simulink model "EL_Model_Simulink"  (R2022a)
settings: Solver=ode5  StartTime=0.0  StopTime=1  FixedStep=0.001  RelTol=1e-3
values from neighbouring files (symbols this model uses):
  a_joint = 160/180*pi    (= 2.79252680319)    [EL_Model_Activation.m]    (also in Form_Finding_Activation.m)
  C_damping = 150    [EL_Model_Activation.m]
  Gt = g'*G    [EL_Model_Activation.m]
  k_cable = 1200    [EL_Model_Activation.m]    (also in Form_Finding_Activation.m)
  k_joint = 35    [EL_Model_Activation.m]    (also in Form_Finding_Activation.m)
  l_cable = sqrt(6)/4*l_leg*sin(a_joint/2)*(1 - delta)    [EL_Model_Activation.m]    (also in Form_Finding_Activation.m = sqrt(6)/4*l_bar*sin(a_joint/2)*(1 - delta))
  l_leg = 0.30    (= 0.3)    [EL_Model_Activation.m]
  m_leg = density*(l_leg*pi*radius^2)+ m_motor + m_battery    (= 0.662767695314)    [EL_Model_Activation.m]
  mu_k = 0.4    [EL_Model_Activation.m]
  mu_s = 0.45    [EL_Model_Activation.m]
  nu_s = 0.25    [EL_Model_Activation.m]
  radius = 0.005    [EL_Model_Activation.m]
  T_damping = 10    [EL_Model_Activation.m]
  X = zeros(36,36,6)    [EL_Model_Activation.m]
  Xbark = zeros(3,36,6)    [EL_Model_Activation.m]
  Xk = zeros(3,36,6)    [EL_Model_Activation.m]
  Y = zeros(36,36,24)    [EL_Model_Activation.m]
  Yk = zeros(3,36,24)    [EL_Model_Activation.m]
settings Model: Creator=LZY-ALIENWARE15  LastModifiedBy=S2974177
settings SolverCC: ExtrapolationOrder=3  AlgebraicLoopSolver=TrustRegion
settings DebuggingCC: UnconnectedInputMsg=warning  UnconnectedOutputMsg=warning  UnconnectedLineMsg=warning  SFMachineParentedDataDiag=warning  UnderSpecifiedDimensionMsg=warning
settings RTWCC: DLArmComputeVersion=19.05

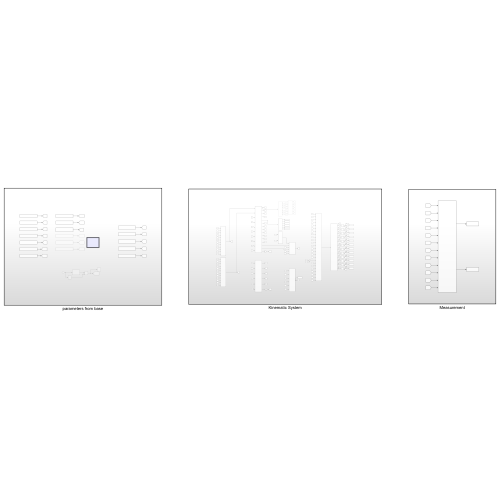
[thumbnail: Simulink's stored preview of the top-level diagram]
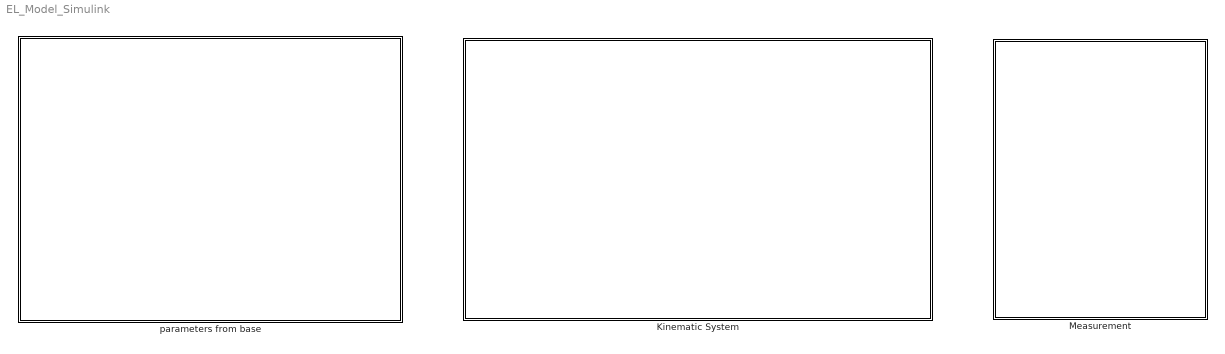
== system EL_Model_Simulink ==
  Kinematic System : Subsystem
  Measurement : Subsystem
  parameters from base : Subsystem

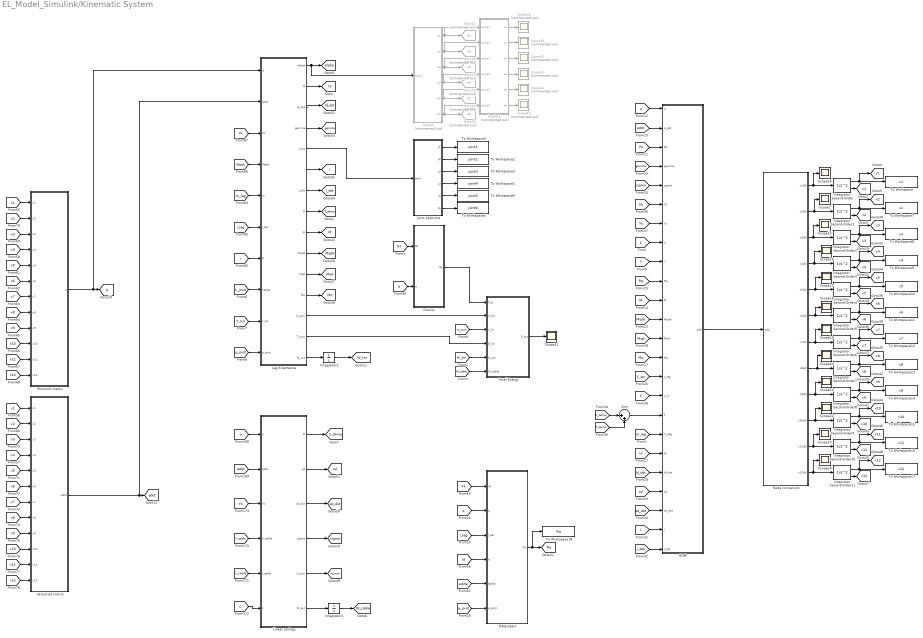
== system EL_Model_Simulink/Kinematic System ==
  Angles : MATLAB Function  Commented=on  TreatAsAtomicUnit=on
  Angles1 : MATLAB Function  Commented=on  TreatAsAtomicUnit=on
  D'Alembert : MATLAB Function  TreatAsAtomicUnit=on
  EOM : MATLAB Function  TreatAsAtomicUnit=on
  Goto13 : Goto  Commented=on  GotoTag=a1  TagVisibility=global
  Goto14 : Goto  Commented=on  GotoTag=a2  TagVisibility=global
  Goto15 : Goto  Commented=on  GotoTag=a3  TagVisibility=global
  Goto16 : Goto  Commented=on  GotoTag=a4  TagVisibility=global
  Goto17 : Goto  Commented=on  GotoTag=a5  TagVisibility=global
  Goto18 : Goto  Commented=on  GotoTag=a6  TagVisibility=global
  Gravity : MATLAB Function  TreatAsAtomicUnit=on
  "Integrator, Second-Order" : SecondOrderIntegrator  ICX=x1_ini  ICDXDT=v1_ini
  "Integrator, Second-Order1" : SecondOrderIntegrator  ICX=x2_ini  ICDXDT=v2_ini
  "Integrator, Second-Order10" : SecondOrderIntegrator  ICX=x11_ini  ICDXDT=v11_ini
  "Integrator, Second-Order11" : SecondOrderIntegrator  ICX=x12_ini  ICDXDT=v12_ini
  "Integrator, Second-Order2" : SecondOrderIntegrator  ICX=x3_ini  ICDXDT=v3_ini
  "Integrator, Second-Order3" : SecondOrderIntegrator  ICX=x4_ini  ICDXDT=v4_ini
  "Integrator, Second-Order4" : SecondOrderIntegrator  ICX=x5_ini  ICDXDT=v5_ini
  "Integrator, Second-Order5" : SecondOrderIntegrator  ICX=x6_ini  ICDXDT=v6_ini
  "Integrator, Second-Order6" : SecondOrderIntegrator  ICX=x7_ini  ICDXDT=v7_ini
  "Integrator, Second-Order7" : SecondOrderIntegrator  ICX=x8_ini  ICDXDT=v8_ini
  "Integrator, Second-Order8" : SecondOrderIntegrator  ICX=x9_ini  ICDXDT=v9_ini
  "Integrator, Second-Order9" : SecondOrderIntegrator  ICX=x10_ini  ICDXDT=v10_ini
  Integrator1 : Integrator
  Integrator2 : Integrator
  Joint positions : MATLAB Function  TreatAsAtomicUnit=on
  Leg Kinematics : MATLAB Function  TreatAsAtomicUnit=on
  Linear springs : MATLAB Function  TreatAsAtomicUnit=on
  Node conversion : MATLAB Function  TreatAsAtomicUnit=on
  Positions matrix : MATLAB Function  TreatAsAtomicUnit=on
  Scope{2,11,14..24} (13 alike) : Scope
  Scope{38..43} (6 alike) : Scope  Commented=on
  Sum : Sum  Inputs=|++
  To Workspace : ToWorkspace  VariableName=x1  SaveFormat=Timeseries  SampleTime=-1
  To Workspace1 : ToWorkspace  VariableName=joint4  SaveFormat=Timeseries  SampleTime=-1
  To Workspace10 : ToWorkspace  VariableName=x5  SaveFormat=Timeseries  SampleTime=-1
  To Workspace11 : ToWorkspace  VariableName=x6  SaveFormat=Timeseries  SampleTime=-1
  To Workspace12 : ToWorkspace  VariableName=x7  SaveFormat=Timeseries  SampleTime=-1
  To Workspace13 : ToWorkspace  VariableName=x8  SaveFormat=Timeseries  SampleTime=-1
  To Workspace14 : ToWorkspace  VariableName=x9  SaveFormat=Timeseries  SampleTime=-1
  To Workspace15 : ToWorkspace  VariableName=x10  SaveFormat=Timeseries  SampleTime=-1
  To Workspace16 : ToWorkspace  VariableName=x11  SaveFormat=Timeseries  SampleTime=-1
  To Workspace17 : ToWorkspace  VariableName=x12  SaveFormat=Timeseries  SampleTime=-1
  To Workspace18 : ToWorkspace  VariableName=Rq  SaveFormat=Timeseries  SampleTime=-1
  To Workspace2 : ToWorkspace  VariableName=joint2  SaveFormat=Timeseries  SampleTime=-1
  To Workspace3 : ToWorkspace  VariableName=joint3  SaveFormat=Timeseries  SampleTime=-1
  To Workspace4 : ToWorkspace  VariableName=joint1  SaveFormat=Timeseries  SampleTime=-1
  To Workspace5 : ToWorkspace  VariableName=joint6  SaveFormat=Timeseries  SampleTime=-1
  To Workspace6 : ToWorkspace  VariableName=joint5  SaveFormat=Timeseries  SampleTime=-1
  To Workspace7 : ToWorkspace  VariableName=x2  SaveFormat=Timeseries  SampleTime=-1
  To Workspace8 : ToWorkspace  VariableName=x3  SaveFormat=Timeseries  SampleTime=-1
  To Workspace9 : ToWorkspace  VariableName=x4  SaveFormat=Timeseries  SampleTime=-1
  Total Energy : MATLAB Function  TreatAsAtomicUnit=on
  Velocities matrix : MATLAB Function  TreatAsAtomicUnit=on
  tag scope: C_damp=global, I=global, I_dot=global, M=global, Mq=global, Mqd=global, Mqdd=global, Rq=global, T_damp=global, Vc_sum=global, W_cable=global, W_tor=global, alpha=global, gamma=global, ld=global, ld_dot=global, q=global, qdot=global, sd=global, sd_dot=global, sigma=global, v10=global, v11=global, v12=global, v1=global, v2=global, v3=global, v4=global, v5=global, v6=global, v7=global, v8=global, v9=global, x10=global, x11=global, x12=global, x1=global, x2=global, x3=global, x4=global, x5=global, x6=global, x7=global, x8=global, x9=global
  wires:
  [qdot] -> Linear springs/2(qdot)
  [Yk] -> Linear springs/3(Yk)
  [v7] -> Velocities matrix/7(v7)
  [x3] -> Positions matrix/3(x3)
  Joint positions/6(j6) -> To Workspace5/1
  [q] -> Linear springs/1(q)
  Angles/2(a2) -> Angles1/2(alpha2), Goto14/1
  [v10] -> Velocities matrix/10(v10)
  [C] -> Linear springs/6(c)
  Angles/6(a6) -> Angles1/6(alpha6), Goto18/1
  Joint positions/1(j1) -> To Workspace4/1
  Gravity/1(Vg) -> Total Energy/1(V_g)
  Angles/5(a5) -> Angles1/5(alpha5), Goto17/1
  Joint positions/2(j2) -> To Workspace2/1
  [x12] -> Positions matrix/12(x12)
  [m_leg] -> Leg Kinematics/5(m)
  [v6] -> Velocities matrix/6(v6)
  [v4] -> Velocities matrix/4(v4)
  [r] -> Leg Kinematics/7(R)
  [l_leg] -> Leg Kinematics/6(l_bar)
  [q] -> Gravity/2(q)
  Linear springs/5(V_sum) -> [Vc_sum]
  [x2] -> Positions matrix/2(x2)
  [v3] -> Velocities matrix/3(v3)
  Angles/4(a4) -> Angles1/4(alpha4), Goto16/1
  Angles/3(a3) -> Angles1/3(alpha3), Goto15/1
  Leg Kinematics/1(alpha) -> [alpha], Angles/1(alpha)
  [Xk] -> Leg Kinematics/3(Xk)
  Angles/1(a1) -> Goto13/1, Angles1/1(alpha1)
  [x5] -> Positions matrix/5(x5)
  Joint positions/3(j3) -> To Workspace3/1
  [Xbark] -> Leg Kinematics/4(Xbark)
  Leg Kinematics/5(joint) -> Joint positions/1(joint)
  Velocities matrix/1(qdot) -> Leg Kinematics/2(qdot), [qdot]
  [v11] -> Velocities matrix/11(v11)
  Positions matrix/1(q) -> Leg Kinematics/1(q), [q]
  [v9] -> Velocities matrix/9(v9)
  [l_cable] -> Linear springs/5(l_cable)
  [v8] -> Velocities matrix/8(v8)
  [v1] -> Velocities matrix/1(v1)
  [x6] -> Positions matrix/6(x6)
  [x1] -> Positions matrix/1(x1)
  [x7] -> Positions matrix/7(x7)
  [v5] -> Velocities matrix/5(v5)
  [x8] -> Positions matrix/8(x8)
  [k_cable] -> Linear springs/4(k_cable)
  [x11] -> Positions matrix/11(x11)
  [v2] -> Velocities matrix/2(v2)
  [v12] -> Velocities matrix/12(v12)
  Joint positions/5(j5) -> To Workspace6/1
  [x4] -> Positions matrix/4(x4)
  [x10] -> Positions matrix/10(x10)
  [x9] -> Positions matrix/9(x9)
  Joint positions/4(j4) -> To Workspace1/1
  Linear springs/1(D) -> [C_damp]
  Leg Kinematics/13(U_sum) -> Total Energy/2(V_tor)
  [C_tor] -> Leg Kinematics/9(c_tor)
  [k_joint] -> Leg Kinematics/8(kappa)
  [a_joint] -> Leg Kinematics/10(a_joint)
  [Vc_sum] -> Total Energy/3(V_lin)
  Total Energy/1(E_tot) -> Scope11/1
  Leg Kinematics/15(W_out) -> Integrator2/1
  Integrator1/1 -> [W_cable]
  Integrator2/1 -> [W_tor]
  Leg Kinematics/9(M) -> [M]
  [W_tor] -> Total Energy/5(W_tor)
  [W_cable] -> Total Energy/6(W_cable)
  Leg Kinematics/14(T_sum) -> Total Energy/4(E_kin)
  [Gt] -> Gravity/1(Gt)
  [X] -> EOM/8(X)
  [Y] -> EOM/9(Y)
  [sigma] -> EOM/5(sigma)
  Linear springs/4(sigma) -> [sigma]
  [Gt] -> EOM/3(Gt)
  [q] -> EOM/1(q)
  [qdot] -> EOM/2(q_dot)
  [M] -> EOM/11(M)
  Leg Kinematics/10(Mqdd) -> [Mqdd]
  Leg Kinematics/11(Mqd) -> [Mqd]
  Leg Kinematics/12(Mq) -> [Mq]
  [Mq] -> EOM/14(Mq)
  [Mqd] -> EOM/13(Mqd)
  [Mqdd] -> EOM/12(Mqdd)
  [Rq] -> EOM/10(Rq)
  Leg Kinematics/2(ld) -> [ld]
  Leg Kinematics/8(D) -> [T_damp]
  Linear springs/3(sd_dot) -> [sd_dot]
  Linear springs/2(sd) -> [sd]
  Leg Kinematics/3(ld_dot) -> [ld_dot]
  Leg Kinematics/4(gamma) -> [gamma]
  Leg Kinematics/7(I_dot) -> [I_dot]
  Leg Kinematics/6(I) -> [I]
  [m_leg] -> EOM/18(m_leg)
  [I_dot] -> EOM/24(I_dot)
  [I] -> EOM/23(I)
  [sd_dot] -> EOM/22(sd_dot)
  [sd] -> EOM/21(sd)
  [ld_dot] -> EOM/20(ld_dot)
  [ld] -> EOM/19(ld)
  [gamma] -> EOM/4(gamma)
  [C] -> EOM/16(c_lin)
  [C_tor] -> EOM/15(c_leg)
  [C_damp] -> Sum/1
  [T_damp] -> Sum/2
  Sum/1 -> EOM/17(f)
  [Xk] -> EOM/6(Xk)
  [Yk] -> EOM/7(Yk)
  Angles1/1(a1) -> Scope38/1
  Angles1/2(a2) -> Scope39/1
  Angles1/3(a3) -> Scope40/1
  Angles1/4(a4) -> Scope41/1
  Angles1/5(a5) -> Scope42/1
  Angles1/6(a6) -> Scope43/1
  Linear springs/6(W_out) -> Integrator1/1
  "Integrator, Second-Order10"/2 -> [v11]
  "Integrator, Second-Order9"/1 -> [x10], To Workspace15/1
  "Integrator, Second-Order5"/1 -> [x6], To Workspace11/1
  "Integrator, Second-Order5"/2 -> [v6]
  "Integrator, Second-Order10"/1 -> [x11], To Workspace16/1
  "Integrator, Second-Order8"/1 -> [x9], To Workspace14/1
  "Integrator, Second-Order4"/2 -> [v5]
  "Integrator, Second-Order7"/1 -> [x8], To Workspace13/1
  "Integrator, Second-Order2"/1 -> [x3], To Workspace8/1
  "Integrator, Second-Order1"/1 -> [x2], To Workspace7/1
  "Integrator, Second-Order3"/2 -> [v4]
  Node conversion/2(x2dd) -> "Integrator, Second-Order1"/1, Scope2/1
  "Integrator, Second-Order"/2 -> [v1]
  "Integrator, Second-Order1"/2 -> [v2]
  Node conversion/9(x9dd) -> Scope21/1, "Integrator, Second-Order8"/1
  Node conversion/10(x10dd) -> Scope22/1, "Integrator, Second-Order9"/1
  "Integrator, Second-Order"/1 -> [x1], To Workspace/1
  Node conversion/8(x8dd) -> Scope20/1, "Integrator, Second-Order7"/1
  Node conversion/3(x3dd) -> Scope15/1, "Integrator, Second-Order2"/1
  "Integrator, Second-Order3"/1 -> [x4], To Workspace9/1
  Node conversion/4(x4dd) -> Scope16/1, "Integrator, Second-Order3"/1
  "Integrator, Second-Order7"/2 -> [v8]
  "Integrator, Second-Order9"/2 -> [v10]
  Node conversion/7(x7dd) -> Scope19/1, "Integrator, Second-Order6"/1
  "Integrator, Second-Order8"/2 -> [v9]
  Node conversion/5(x5dd) -> Scope17/1, "Integrator, Second-Order4"/1
  "Integrator, Second-Order4"/1 -> [x5], To Workspace10/1
  "Integrator, Second-Order2"/2 -> [v3]
  "Integrator, Second-Order11"/1 -> [x12], To Workspace17/1
  Node conversion/1(x1dd) -> Scope14/1, "Integrator, Second-Order"/1
  "Integrator, Second-Order6"/2 -> [v7]
  Node conversion/12(x12dd) -> "Integrator, Second-Order11"/1, Scope24/1
  "Integrator, Second-Order11"/2 -> [v12]
  Node conversion/11(x11dd) -> Scope23/1, "Integrator, Second-Order10"/1
  Node conversion/6(x6dd) -> Scope18/1, "Integrator, Second-Order5"/1
  "Integrator, Second-Order6"/1 -> [x7], To Workspace12/1
  EOM/1(qdd) -> Node conversion/1(qdd)
  [q] -> D'Alembert/2(q)
  [a_joint] -> D'Alembert/6(a_joint)
  [alpha] -> D'Alembert/5(alpha)
  [l_leg] -> D'Alembert/3(l_bar)
  [ld] -> D'Alembert/4(d)
  D'Alembert/1(Rq) -> To Workspace18/1, [Rq]
  [Xk] -> D'Alembert/1(Xk)

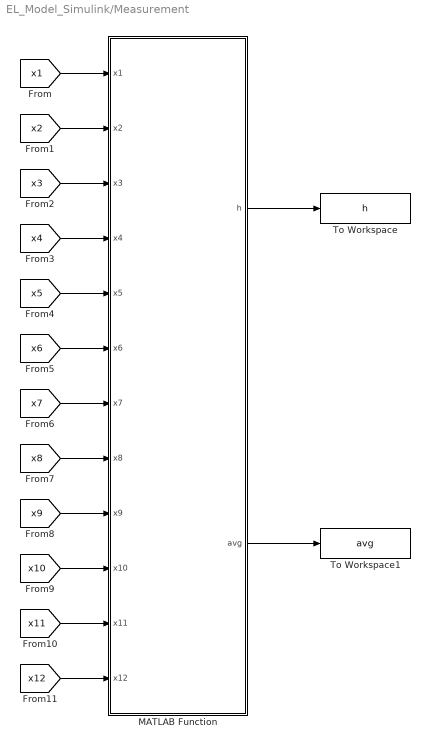
== system EL_Model_Simulink/Measurement ==
  MATLAB Function : MATLAB Function  TreatAsAtomicUnit=on
  To Workspace : ToWorkspace  VariableName=h  SaveFormat=Timeseries  SampleTime=-1
  To Workspace1 : ToWorkspace  VariableName=avg  SaveFormat=Timeseries  SampleTime=-1
  wires:
  [x1] -> MATLAB Function/1(x1)
  [x2] -> MATLAB Function/2(x2)
  [x3] -> MATLAB Function/3(x3)
  [x4] -> MATLAB Function/4(x4)
  [x5] -> MATLAB Function/5(x5)
  [x6] -> MATLAB Function/6(x6)
  [x8] -> MATLAB Function/8(x8)
  [x9] -> MATLAB Function/9(x9)
  [x10] -> MATLAB Function/10(x10)
  [x11] -> MATLAB Function/11(x11)
  [x12] -> MATLAB Function/12(x12)
  [x7] -> MATLAB Function/7(x7)
  MATLAB Function/1(h) -> To Workspace/1
  MATLAB Function/2(avg) -> To Workspace1/1

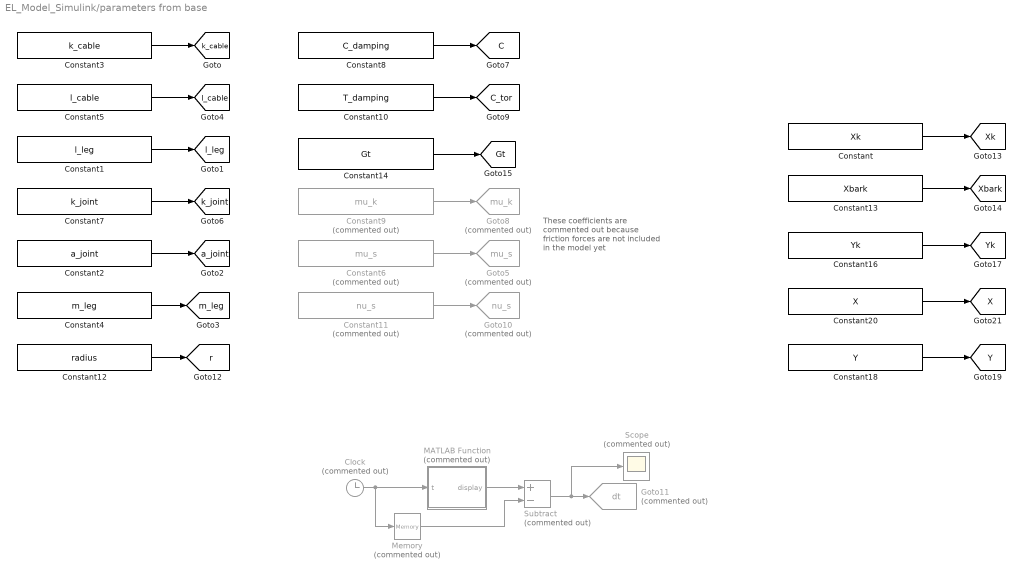
== system EL_Model_Simulink/parameters from base ==
  note: These coefficients
      | are commented
      | out because friction
      | forces are not
      | included in the
      | model yet
  Clock : Clock  Commented=on
  Constant : Constant  Value=Xk  VectorParams1D=off
  Constant1 : Constant  Value=l_leg
  Constant10 : Constant  Value=T_damping
  Constant11 : Constant  Commented=on  Value=nu_s
  Constant12 : Constant  Value=radius
  Constant13 : Constant  Value=Xbark  VectorParams1D=off
  Constant14 : Constant  Value=Gt
  Constant16 : Constant  Value=Yk  VectorParams1D=off
  Constant18 : Constant  Value=Y  VectorParams1D=off
  Constant2 : Constant  Value=a_joint
  Constant20 : Constant  Value=X  VectorParams1D=off
  Constant3 : Constant  Value=k_cable
  Constant4 : Constant  Value=m_leg
  Constant5 : Constant  Value=l_cable
  Constant6 : Constant  Commented=on  Value=mu_s
  Constant7 : Constant  Value=k_joint
  Constant8 : Constant  Value=C_damping
  Constant9 : Constant  Commented=on  Value=mu_k
  Goto10 : Goto  Commented=on  GotoTag=nu_s  TagVisibility=global
  Goto11 : Goto  Commented=on  GotoTag=dt  TagVisibility=global
  Goto5 : Goto  Commented=on  GotoTag=mu_s  TagVisibility=global
  Goto8 : Goto  Commented=on  GotoTag=mu_k  TagVisibility=global
  MATLAB Function : MATLAB Function  Commented=on  TreatAsAtomicUnit=on
  Memory : Memory  Commented=on
  Scope : Scope  Commented=on
  Subtract : Sum  Commented=on  Inputs=+-
  tag scope: C=global, C_tor=global, Gt=global, X=global, Xbark=global, Xk=global, Y=global, Yk=global, a_joint=global, k_cable=global, k_joint=global, l_cable=global, l_leg=global, m_leg=global, r=global
  wires:
  Constant3/1 -> [k_cable]
  Constant1/1 -> [l_leg]
  Constant5/1 -> [l_cable]
  Constant7/1 -> [k_joint]
  Constant2/1 -> [a_joint]
  Constant4/1 -> [m_leg]
  Constant8/1 -> [C]
  Constant9/1 -> Goto8/1
  Constant10/1 -> [C_tor]
  Constant6/1 -> Goto5/1
  Constant11/1 -> Goto10/1
  Subtract/1 -> Scope/1, Goto11/1
  Memory/1 -> Subtract/2
  Constant12/1 -> [r]
  Constant/1 -> [Xk]
  Constant13/1 -> [Xbark]
  Constant14/1 -> [Gt]
  Constant16/1 -> [Yk]
  Constant18/1 -> [Y]
  Constant20/1 -> [X]
  MATLAB Function/1(display) -> Subtract/1
  Clock/1 -> MATLAB Function/1(t), Memory/1

== matlab function EL_Model_Simulink/Kinematic System/D'Alembert ==
  data: Xk input; q input; l_bar input; d input; alpha input; a_joint input; Rq output
function Rq = leg_constraint(Xk,q,l_bar,d,alpha,a_joint)
% Empty matrices and vector to be filled in
Rq = zeros(30,36);
exponent = zeros(1,6);

% Parameter that influences steepness of the walls of the potential well
p = 10^3;

% Term in front of the exponent
coeff = (2-4/l_bar^2)*10^3;

% Inner limit of the joint angle
a_inner = (180-a_joint)*pi/180;

for i = 1:6
    if alpha(i) > a_joint
        exponent(i) = exp(p*(d(i)-norm(l_bar*cos(a_joint))));
    elseif alpha(i) < a_inner
        exponent(i) = exp(-p*(d(i)-norm(l_bar*cos(a_inner))));
    else
        exponent(i) = 0;
    end
    Rq(i+24,:) = coeff*exponent(i)*q'*Xk(:,:,i)'*Xk(:,:,i);
end

end

== matlab function EL_Model_Simulink/Measurement/MATLAB Function ==
  data: x1 input; h output; x2 input; x3 input; x4 input; x5 input; x6 input; x7 input; x8 input; x9 input; x10 input; x11 input; x12 input; avg output
function [h,avg] = measurement(x1,x2,x3,x4,x5,x6,x7,x8,x9,x10,x11,x12)
xz = [x1(3) x2(3) x3(3) x4(3) x5(3) x6(3) x7(3) x8(3) x9(3) x10(3) x11(3) x12(3)];
h = min(xz);


plane_pos = [x1(1:2) x2(1:2) x3(1:2) x4(1:2) x5(1:2) x6(1:2) x7(1:2) x8(1:2) x9(1:2) x10(1:2) x11(1:2) x12(1:2)];

avg = [sum(plane_pos(1,:))/12 ; sum(plane_pos(2,:))/12];



end

== matlab function EL_Model_Simulink/Kinematic System/Positions matrix ==
  data: x1 input; q output; x2 input; x3 input; x4 input; x5 input; x6 input; x7 input; x8 input; x9 input; x10 input; x11 input; x12 input
function q = q_vector(x1,x2,x3,x4,x5,x6,x7,x8,x9,x10,x11,x12)
% Concatenation of position vctors into one 36x1 vector q
q = [x1 ;x2 ;x3 ;x4 ;x5 ;x6 ;x7 ;x8; x9 ;x10; x11; x12];

== matlab function EL_Model_Simulink/Kinematic System/Velocities matrix ==
  data: v1 input; qdot output; v2 input; v3 input; v4 input; v5 input; v6 input; v7 input; v8 input; v9 input; v10 input; v11 input; v12 input
function qdot = qdot_vector(v1,v2,v3,v4,v5,v6,v7,v8,v9,v10,v11,v12)
% Concatenation of position vctors into one 36x1 vector qdot
qdot = [v1 ;v2 ;v3 ;v4 ;v5 ;v6 ;v7 ;v8 ;v9 ;v10 ;v11 ;v12];

== matlab function EL_Model_Simulink/Kinematic System/Total Energy ==
  data: V_g input; E_tot output; V_tor input; V_lin input; E_kin input; W_tor input; W_cable input
function E_tot = total_energy(V_g,V_tor,V_lin,E_kin, W_tor, W_cable)
% Sum of potential energy, kinetic energy and work done by the damping
% dissipation forces
E_tot = E_kin + V_g + V_tor + V_lin + W_tor + W_cable;

end

== matlab function EL_Model_Simulink/Kinematic System/Leg Kinematics ==
  data: alpha output; q input; qdot input; Xk input; Xbark input; ld output; ld_dot output; gamma output; joint output; I output; I_dot output; D output; M output; Mqdd output; Mqd output; Mq output; U_sum output; T_sum output; m input; l_bar input; R input; W_out output; kappa input; c_tor input; a_joint input
function [alpha,ld,ld_dot,gamma,joint,I,I_dot,D,M,Mqdd,Mqd,Mq,U_sum,T_sum,W_out] = leg_kinematics(q,qdot,Xk,Xbark, m, l_bar, R, kappa, c_tor, a_joint)
% Empty matrices and vector to be filled in
b = zeros(3,6);
b_b = zeros(3,6);
v_b = zeros(3,6);
v_diff = zeros(3,6);
mag = zeros(1,6);
L = zeros(1,6);
ld_dot = zeros(1,6);
ld = zeros(1,6); %
alpha = zeros(1,6); %
p = zeros(1,6); %

% Vectors used for joint plotting
normal = zeros(6,3); % Watch the reversed order of dimensions!
b_norm = zeros(6,3);
NOR = zeros(6,3);
X = zeros(6,3);

% Inertia and angular momentum
omega = zeros(3,6);
I = zeros(1,6);
I_dot = zeros(1,6);

% A series of mass matrices and their derivatives
M = zeros(36,36,6);
M_dot = zeros(36,36,6);
Mf = zeros(36,36,6);
Mqdd = zeros(36,36,6);
Mqd = zeros(36,36,6);
Mq = zeros(36,36,6);
F = zeros(36,36,6);

damp_mag = zeros(6,1);

h_k = zeros(3,6);

T = zeros(1,6);
T_f = zeros(1,6);

Rot = zeros(6,3);
joint = zeros(3,6);
v_joint = zeros(3,6);
v_b_bar = zeros(3,6);

gamma = zeros(6,1);
U = zeros(6,1);
damp = zeros(3,6);
D = zeros(36,1);
W_int = zeros(6,1);

Q = zeros(6,1);

x_3rd = [q(16:18) q(10:12) q(13:15) q(4:6) q(7:9) q(1:3)]; % 3x6 matrix


for i = 1:6
    % Leg connected node separation, velocities, etc.
    b(:,i) = Xk(:,:,i)*q; % Leg vector
    L(i) = dot(b(:,i),b(:,i)); % = l_bk^2
    b_b(:,i) = Xbark(:,:,i)*q; % Leg COM vector
    v_diff(:,i) = Xk(:,:,i)*qdot; % Relative velocity of connected nodes
    v_b(:,i) = Xbark(:,:,i)*qdot; % velocity of the COM

    % Distance between the end nodes
    ld(i) = norm(b(:,i)); % Norm of node separation
    mag(i) = (l_bar^2-2*ld(i)^2)/(l_bar^2);
    alpha(i) = acos(mag(i)); % Angle
    ld_dot(i) = b(:,i)'*v_diff(:,i)/ld(i); % Change in end-node separation for a compressible bar
    
    % Joint distance from central axis
    p(i) = l_bar/2*cos(alpha(i)/2); % vector
    
    % Joint position preparation
    k = 3*i; % Index used for easier notation in next equation
    normal(i,:) = cross(transpose(-b(:,i)),transpose(q(k-2:k)-x_3rd(:,i))); % 3x6 matrix
    
    % Rotating a vector 90 degrees for the direction of the joint
    b_norm(i,:) = transpose(b(:,i)/ld(i)); % 3x6 matrix
    NOR(i,:) = normal(i,:)/norm(normal(i,:)); % 3x6 matrix
    X(i,:) = cross(b_norm(i,:),NOR(i,:)); % 3x6 matrix 
    Rot(i,:) = cross(b_norm(i,:),NOR(i,:));
    joint(:,i) = p(i) * transpose(Rot(i,:)) + b_b(:,i); % 3x6 matrix: Joint positions

    % Joint velocities
    Q(i) = sign(dot(v_diff(:,i),b_norm(i,:))); % Determine if nodes are moving closer or moving apart
    v_joint(:,i) = transpose(X(i,:))*Q(i)*norm(v_diff(:,i))/(2*tan(alpha(i)/2)); % Velocity of the joint
    v_b_bar(:,i) = v_b(:,i) + v_joint(:,i); % Velocity of the center of mass
    
    % Inertia and angular momentum
    omega(:,i) = (cross(b(:,i),v_diff(:,i)))/L(i); % 3x6 matrix: Angular velocities
    I(i) = m*(3*R^2 + ld(i)^2)/(12*ld(i)^2); % 1x6 vector: Moments of Inertia
    I_dot(i) = m*ld(i)*ld_dot(i)/6; % 1x6 vector: Time derivative of I(i);
    h_k(:,i) = I(i) * omega(:,i); % 3x6 matrix: Angular momenta
    
    % Mass matrices, with their derivatives that depend on changing bar
    % length among others. All of them are 36x36 matrices    
    F(:,:,i) = 1/ld(i)^3 * Xk(:,:,i)'*Xk(:,:,i);    % Matrix F is used for as a substitute in following equations

    M(:,:,i) = m*Xbark(:,:,i)'*Xbark(:,:,i) + I(i)/L(i)*Xk(:,:,i)'*Xk(:,:,i);
    Mf(:,:,i) = I(i)*F(:,:,i)*ld_dot(i);
    M_dot(:,:,i) = I_dot(i)/(L(i))*Xk(:,:,i)'*Xk(:,:,i) - 2 * Mf(:,:,i);
    
    Mqdd(:,:,i) = M(:,:,i) - Xk(:,:,i)'*Xk(:,:,i)*q/norm(b(:,i)) * I(i)*q'*F(:,:,i);
    Mqd(:,:,i) = M_dot(:,:,i) - Mf(:,:,i);
    Mq(:,:,i) = -I_dot(i)*F(:,:,i)*ld_dot(i) + 3*I(i)*F(:,:,i)*ld_dot(i)^2/ld(i) - (qdot'*Xk(:,:,i)'*Xk(:,:,i)*qdot/ld(i) - (q'*Xk(:,:,i)'*Xk(:,:,i)*qdot)/L(i)*ld_dot(i))*I(i)*F(:,:,i);
    
    % Kinetic energies
    T_f(i) = 0.5 * I(i)/L(i) * ld_dot(i)^2;
    T(i) = 0.5*qdot'*M(:,:,i)*qdot - T_f(i);
    
    % Damping
    damp_mag(i) = -c_tor*(v_diff(:,i)'*b(:,i))/ld(i);
    damp(:,i) = -c_tor*(v_diff(:,i)'*b(:,i))/ld(i) * (b(:,i)/ld(i));
    
    D = D + Xk(:,:,i)'*damp(:,i); % Damping magnitude in a leg
    
    % Force density of torsion spring
    if alpha(i) < a_joint
        gamma(i) = 4*kappa*(alpha(i)-a_joint)/(sqrt(1-mag(i)^2));
    end
    % Potential energy and work
    U(i) = 0.5 * kappa * (alpha(i) - a_joint)^2;
    W_int(i) = dot(damp(:,i),v_diff(:,i));
end

U_sum = sum(U);
T_sum = sum(T);
W_out = sum(W_int);

end

== matlab function EL_Model_Simulink/Kinematic System/Gravity ==
  data: Gt input; Vg output; q input
function Vg = gravity(Gt,q)

Vg= -Gt'*q;

end

== matlab function EL_Model_Simulink/Kinematic System/Angles ==
  data: alpha input; a1 output; a2 output; a3 output; a4 output; a5 output; a6 output
function [a1,a2,a3,a4,a5,a6] = angles(alpha)
a1 = alpha(1);
a2 = alpha(2);
a3 = alpha(3);
a4 = alpha(4);
a5 = alpha(5);
a6 = alpha(6);
end

== matlab function EL_Model_Simulink/Kinematic System/Joint positions ==
  data: joint input; j1 output; j2 output; j3 output; j4 output; j5 output; j6 output
function [j1,j2,j3,j4,j5,j6] = joints(joint)
j1 = joint(:,1);
j2 = joint(:,2);
j3 = joint(:,3);
j4 = joint(:,4);
j5 = joint(:,5);
j6 = joint(:,6);
end

== matlab function EL_Model_Simulink/Kinematic System/EOM ==
  data: q input; q_dot input; Gt input; gamma input; sigma input; Xk input; Yk input; X input; Y input; Rq input; M input; Mqdd input; Mqd input; Mq input; c_leg input; c_lin input; f input; m_leg input; ld input; ld_dot input; sd input; sd_dot input; I input; I_dot input; qdd output
function qdd = EOM(q,q_dot,Gt,gamma,sigma,Xk,Yk,X,Y,Rq,M,Mqdd,Mqd,Mq,c_leg,c_lin,f,m_leg,ld,ld_dot,sd,sd_dot,I,I_dot)
% Empty matrices and vector to be filled in
dVs = zeros(36,1);
dVl = zeros(36,1);
M_inv = zeros(36,36);
Mq_sum = zeros(36,36);
Mqd_sum = zeros(36,36);
Mqdd_sum = zeros(36,36);

term1 = zeros(36,36);
term2 = zeros(36,36);

% Bar length derivatives w.r.t. q
dl_bk = zeros(6,36);
dldot_bk = zeros(6,36);

% Cable length derivatives
dl_sk = zeros(24,36);
dldot_sk = zeros(24,36);

% Inertia derivatives w.r.t. q
dI_bk = zeros(6,36);
dIdot_bk = zeros(6,36);
dIdot_dqdot = zeros(6,36);

% Damping of springs and legs
dfl_dq = zeros(3,36,6);
dfs_dq = zeros(3,36,24);
dfl_dq_dot = zeros(3,36,6);
dfs_dq_dot = zeros(3,36,24);

dfl_dq_sum = zeros(36,36);
dfs_dq_sum = zeros(36,36);
dfl_dq_dot_sum = zeros(36,36);
dfs_dq_dot_sum = zeros(36,36);

% Mass matrix derivatives
dMq_dqdot = zeros(36,36,6);
dMqdot_dqdot = zeros(36,36,6);

XX = zeros(36,216);
YY = zeros(36,864);

X_hat = zeros(36,6);
Y_hat = zeros(36,24);

% Gravitational potential energy change (dVg/dq)
dVg = -Gt; %For now, gravity is not implemented any further

% String potential energy change (dVs/dq)
for j = 1:24
    % String potential energy change (dVs/dq)
    dVs = dVs + sigma(j)*Y(:,:,j)*q;

    % Cable length derivatives
    dl_sk(j,:) = q'*Y(:,:,j)/sd(j);
    dldot_sk(j,:) = q_dot'*Y(:,:,j)/sd(j) - (q_dot'*Y(:,:,j)*q/sd(j)^2)*dl_sk(j,:);

    % Damping
    dfs_dq(:,:,j) = -c_lin*(Yk(:,:,j)*q/sd(j)*dldot_sk(j,:) + sd_dot(j)*Yk(:,:,j)/sd(j) - sd_dot(j)*Yk(:,:,j)*q/sd(j)^2 * dl_sk(j,:));
    dfs_dq_dot(:,:,j) = -c_lin*(Yk(:,:,j)*q/sd(j) * dl_sk(j,:));

    dfs_dq_sum = dfs_dq_sum + Yk(:,:,j)'*dfs_dq(:,:,j);
    dfs_dq_dot_sum = dfs_dq_dot_sum + Yk(:,:,j)'*dfs_dq_dot(:,:,j);

    k = j*36;
    YY(:,k-35:k) = Y(:,:,j);

    Y_hat(:,j) = Y(:,:,j)'*q;
end

% Leg potential energy change (dVl/dq)
for i = 1:6
    dVl = dVl + gamma(i)*X(:,:,i)*q;
    M_inv = M_inv + pinv(M(:,:,i));
    
    % Bar length derivatives used in term1
    dl_bk(i,:) = q'*X(:,:,i)/ld(i);
    dldot_bk(i,:) = q_dot'*X(:,:,i)/ld(i) - (q_dot'*X(:,:,i)*q/ld(i)^2)*dl_bk(i,:);

    % Damping
    dfl_dq(:,:,i) = -c_leg*(Xk(:,:,i)*q/ld(i)*dldot_bk(i,:) + ld_dot(i)*Xk(:,:,i)/ld(i) - ld_dot(i)*Xk(:,:,i)*q/ld(i)^2 * dl_bk(i,:));
    dfl_dq_dot(:,:,i) = -c_leg*(Xk(:,:,i)*q/ld(i) * dl_bk(i,:));

    dfl_dq_sum = dfl_dq_sum + Xk(:,:,i)'*dfl_dq(:,:,i);
    dfl_dq_dot_sum = dfl_dq_dot_sum + Xk(:,:,i)'*dfl_dq_dot(:,:,i);
    

    % Inertia derivatives
    dI_bk(i,:) = (m_leg*ld(i))/6*dl_bk(i,:);
    dIdot_bk(i,:) = m_leg/6 * (ld_dot(i)*dl_bk(i,:) + ld(i)*dldot_bk(i,:));
    dIdot_dqdot(i,:) = m_leg/6 * q'*X(:,:,i);

    % Mass matrix derivatives
    dMq_dqdot(:,:,i) = (1/ld(i)^3)*X(:,:,i)*q*ld_dot(i)*dIdot_dqdot(i,:) + I_dot(i)*X(:,:,i)*q/ld(i)^3*dl_bk(i,:) - 6*(I(i)*X(:,:,i)*q*ld_dot(i)/ld(i)^4*dl_bk(i,:) + (I(i)*X(:,:,i)/ld(i)^3)*(2*X(:,:,i)*q*transpose(q_dot)/ld(i) - q*transpose(q)*X(:,:,i)*ld_dot(i)/ld(i)^2) - q*transpose(q)*X(:,:,i)*q_dot/ld(i)^2 * dl_bk(i,:));
    dMqdot_dqdot(:,:,i) = -3*(I(i)/ld(i)^3)*X(:,:,i)*q_dot*dl_bk(i,:) + (1/ld(i)^2)*X(:,:,i)*q_dot*dIdot_dqdot(i,:);

    term1 = term1 + X(:,:,i)*q_dot*(-3*(I(i)/ld(i)^3)*dldot_bk(i,:) - 3*(I(i)*ld_dot(i)/ld(i)^4)*dl_bk(i,:) + 1/ld(i)^2*dIdot_bk(i,:) - 2*I_dot(i)*1/ld(i)^3 *dl_bk(i,:) - 3*ld_dot(i)/ld(i)^3 * dI_bk(i,:)) ; % := dM_qdot^T/dq * qdot for in => (d_ksi3 / dq)*qdot
    term2 = term2 - dMq_dqdot(:,:,i) - transpose(Mqd(:,:,i)) - dMqdot_dqdot(:,:,i);
    
    p = i*36;
    XX(:,p-35:p) = X(:,:,i);

    Mq_sum = Mq_sum + Mq(:,:,i);
    Mqd_sum = Mqd_sum + Mqd(:,:,i);

    Mqdd_sum = Mqdd_sum + Mqdd(:,:,i);

    X_hat(:,i) = X(:,:,i)'*q;
end

%% NONLINEAR DESCRIPTION
Mqdd_inv = pinv(Mqdd_sum);
B = (-(Mq_sum'*q + dVl + dVs) - Mqd_sum'*q_dot + f + Rq'*ones(30,1));  % + Gt 
qdd = Mqdd_inv*B;


%% Variable bar lengths
dampterm1 = dfs_dq_sum + dfl_dq_sum;
dampterm2 = dfs_dq_dot_sum + dfl_dq_dot_sum;

kron_gamma = kron(transpose(gamma),eye(36));
kron_sigma = kron(transpose(sigma),eye(36));

d_ksi_3_dq = (-(transpose(Mq_sum) + kron_gamma*transpose(XX) + kron_sigma*transpose(YY))- term1 + dampterm1);
d_ksi_3_dqdot = (term2 + dampterm2);
d_ksi_3_dgam = X_hat;
d_ksi_3_dsig = -Y_hat;


%% LINEARIZED SYSTEM
% M_alpha = pinv([Mqdd_sum zeros(36,30);
%             zeros(30,36) zeros(30,30)]);
% 
% M_beta = M_alpha(1:36,1:36);
% 
% A = [zeros(36,36)            eye(36);
%      M_beta*d_ksi_3_dq  M_beta*d_ksi_3_dqdot];
% Bu = [zeros(36,24)            zeros(36,6)   ;
%       M_beta*d_ksi_3_dsig  M_beta*d_ksi_3_dgam];
% 
% x = [q;
%     q_dot];
% u = [sigma;
%      gamma];
% 
% xdot = A*x + Bu*u;
% 
% qd = xdot(1:36);
% qdd = xdot(37:72);

end

== matlab function EL_Model_Simulink/Kinematic System/Node conversion ==
  data: qdd input; x1dd output; x2dd output; x3dd output; x4dd output; x5dd output; x6dd output; x7dd output; x8dd output; x9dd output; x10dd output; x11dd output; x12dd output
function [x1dd, x2dd, x3dd, x4dd, x5dd, x6dd, x7dd, x8dd, x9dd, x10dd, x11dd, x12dd] = node_conv(qdd)
% Splitting up the single long vector into 3-dimensional node accelerations
% to be integrated in the blocks right next to this function
x1dd = qdd(1:3);
x2dd = qdd(4:6);
x3dd = qdd(7:9);
x4dd = qdd(10:12);
x5dd = qdd(13:15);
x6dd = qdd(16:18);
x7dd = qdd(19:21);
x8dd = qdd(22:24);
x9dd = qdd(25:27);
x10dd = qdd(28:30);
x11dd = qdd(31:33);
x12dd = qdd(34:36);

end

== matlab function EL_Model_Simulink/parameters from base/MATLAB Function ==
  data: t input; display output
function display = clock(t)
display = t;
end

== matlab function EL_Model_Simulink/Kinematic System/Angles1 ==
  data: alpha1 input; a1 output; a2 output; a3 output; a4 output; a5 output; a6 output; alpha2 input; alpha3 input; alpha4 input; alpha5 input; alpha6 input
function [a1,a2,a3,a4,a5,a6] = angles(alpha1,alpha2,alpha3,alpha4,alpha5,alpha6)
a1 = 180/pi*alpha1;
a2 = 180/pi*alpha2;
a3 = 180/pi*alpha3;
a4 = 180/pi*alpha4;
a5 = 180/pi*alpha5;
a6 = 180/pi*alpha6;
end

== matlab function EL_Model_Simulink/Kinematic System/Linear springs ==
  data: q input; qdot input; Yk input; k_cable input; l_cable input; c input; D output; sd output; sd_dot output; sigma output; V_sum output; W_out output
function [D, sd, sd_dot, sigma, V_sum, W_out]= cables(q,qdot,Yk,k_cable,l_cable,c)
% Empty matrices and vector to be filled in
s_k = zeros(3,24);
v_s = zeros(3,24);
sigma = zeros(24,1);
sd = zeros(24,1);
sd_dot = zeros(24,1);
Vs = zeros(24,1);
damp = zeros(3,24);
D = zeros(36,1);
W_int = zeros(24,1);

%% New code
for i = 1:24
    s_k(:,i) = Yk(:,:,i)*q; % Node separation of cable connected nodes
    sd(i) = norm(s_k(:,i)); % Magnitude
    v_s(:,i) = Yk(:,:,i)*qdot; % Relative velocity of cable connected nodes
    sd_dot(i) = s_k(:,i)'*v_s(:,i)/sd(i); % Velocity magnitude of a node set connected by a cable

    % Only when the cable is in tension there is a non-zero force density
    % in the string
    if sd(i)-l_cable > 0
        sigma(i) = (k_cable*(1 - l_cable/sd(i))); % Force density in a string when in tension
        damp(:,i) = -c*(v_s(:,i)'*s_k(:,i))*s_k(:,i)/sd(i)^2; % Damping vector
        Vs(i) = 0.5*(sigma(i)^2/k_cable)*sd(i)^2; % Potential energy stored in the string
    else
        sigma(i) = 0;
        damp(:,i) = [0;0;0];
        Vs(i) = 0;
    end
    W_int(i) = dot(damp(:,i),v_s(:,i)); % Work done by the damping in the spring
    D = D + Yk(:,:,i)'*damp(:,i); % Damping in individual strings
end
V_sum = sum(Vs);
W_out = sum(W_int);

end
